simulink library "csc_ppc_phase_plane_ctrl_mtv_lib"  (R2014b)
settings: Solver=ode45  StartTime=0.0  StopTime=10.0  RelTol=1e-3
libraries: util_common_lib x2, util_quat_lib x2, util_info_lib x1, csc_cac_coarse_acs_cntrl_mtv_lib x1, csc_vac_vernier_acs_ctrl_lib x1
settings Model: Creator=tgorton  LastModifiedBy=tgorton

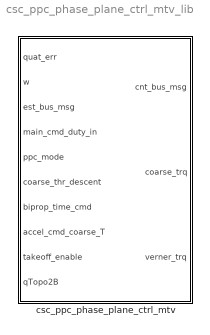
== system csc_ppc_phase_plane_ctrl_mtv_lib ==
  csc_ppc_phase_plane_ctrl_mtv : Subsystem

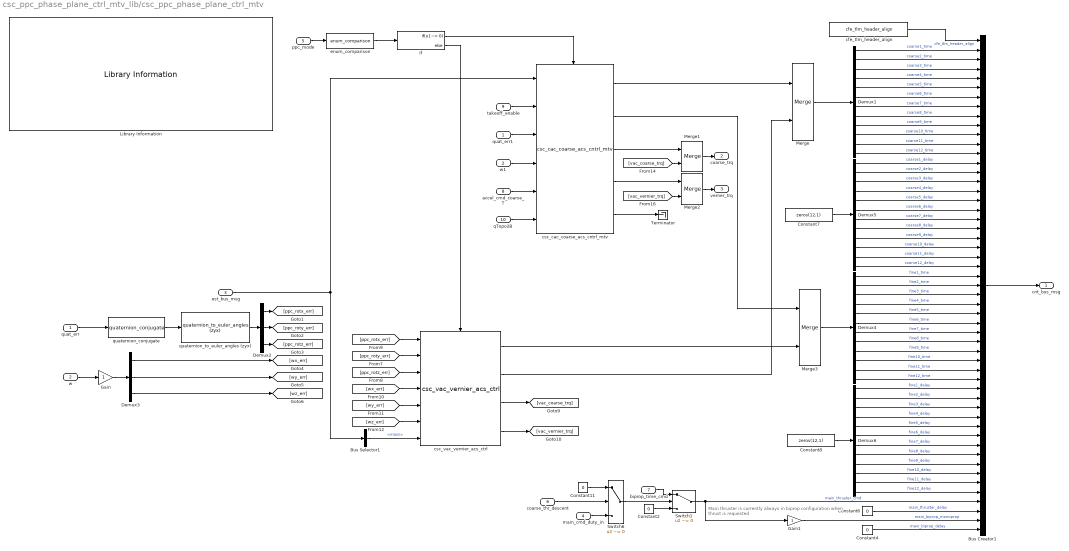
== system csc_ppc_phase_plane_ctrl_mtv_lib/csc_ppc_phase_plane_ctrl_mtv ==
  note: Main thruster is currently always in biprop configuration
      | when thrust is requested
  quat_err : Inport
  w : Inport  Port=2
  est_bus_msg : Inport  Port=3
  main_cmd_duty_in : Inport  Port=4
  ppc_mode : Inport  Port=5
  coarse_thr_descent : Inport  Port=6
  biprop_time_cmd : Inport  Port=7
  accel_cmd_coarse_T : Inport  Port=8
  takeoff_enable : Inport  Port=9
  qTopo2B : Inport  Port=10
  Bus Creator1 : BusCreator  Inputs=53  OutDataTypeStr=Bus: cnt_bus_msg  NonVirtualBus=on
  Bus Selector1 : BusSelector  OutputSignals=mass
  Constant11 : Constant  Value=0  OutDataTypeStr=boolean
  Constant2 : Constant  Value=0  OutDataTypeStr=uint8
  Constant4 : Constant  Value=0  OutDataTypeStr=uint8
  Constant6 : Constant  Value=0  OutDataTypeStr=uint8
  Constant7 : Constant  Value=zeros(12,1)  OutDataTypeStr=uint8
  Constant8 : Constant  Value=zeros(12,1)  OutDataTypeStr=uint8
  Demux{1,4..6} (4 alike) : Demux  Outputs=12
  Demux2 : Demux  Outputs=3
  Demux3 : Demux  Outputs=3
  Gain : Gain
  Gain1 : Gain  OutDataTypeStr=uint8
  If : If  IfExpression=u1~= 0
  Library Information : util_info_lib/Library Information  owner='jkaidy'
  Merge{,1..3} (4 alike) : Merge
  Switch1 : Switch  Criteria=u2 ~= 0
  Switch6 : Switch  Criteria=u2 ~= 0
  Terminator : Terminator
  cfe_tlm_header_align : util_common_lib/cfe_tlm_header_align
  csc_cac_coarse_acs_cntrl_mtv : csc_cac_coarse_acs_cntrl_mtv_lib/csc_cac_coarse_acs_cntrl_mtv
  csc_vac_vernier_acs_ctrl : csc_vac_vernier_acs_ctrl_lib/csc_vac_vernier_acs_ctrl
  enum_comparison : util_common_lib/enum_comparison  comparison_type===
  quat_err1 : InportShadow
  quaternion_conjugate : util_quat_lib/quaternion_conjugate  SystemSampleTime=-1
  quaternion_to_euler_angles (zyx) : util_quat_lib/quaternion_to_euler_angles (zyx)  SystemSampleTime=-1
  w1 : InportShadow  Port=2
  cnt_bus_msg : Outport
  coarse_trq : Outport  Port=2
  verner_trq : Outport  Port=3
  wires:
  quat_err1/1 -> csc_cac_coarse_acs_cntrl_mtv/3
  qTopo2B/1 -> csc_cac_coarse_acs_cntrl_mtv/6
  accel_cmd_coarse_T/1 -> csc_cac_coarse_acs_cntrl_mtv/5
  w1/1 -> csc_cac_coarse_acs_cntrl_mtv/4
  Bus Selector1/1 -> csc_vac_vernier_acs_ctrl/7  "<mass>"
  csc_cac_coarse_acs_cntrl_mtv/1 -> Merge/1
  Demux3/3 -> [wz_err]
  Demux3/2 -> [wy_err]
  Demux3/1 -> [wx_err]
  Gain/1 -> Demux3/1
  est_bus_msg/1 -> Bus Selector1/1, csc_cac_coarse_acs_cntrl_mtv/1
  ppc_mode/1 -> enum_comparison/1
  [ppc_rotx_err] -> csc_vac_vernier_acs_ctrl/1
  [ppc_roty_err] -> csc_vac_vernier_acs_ctrl/2
  [ppc_rotz_err] -> csc_vac_vernier_acs_ctrl/3
  [wz_err] -> csc_vac_vernier_acs_ctrl/6
  [wx_err] -> csc_vac_vernier_acs_ctrl/4
  [wy_err] -> csc_vac_vernier_acs_ctrl/5
  w/1 -> Gain/1
  quat_err/1 -> quaternion_conjugate/1
  biprop_time_cmd/1 -> Switch1/1
  Constant2/1 -> Switch1/3
  coarse_thr_descent/1 -> Switch6/2
  main_cmd_duty_in/1 -> Switch6/3
  Constant11/1 -> Switch6/1
  Switch6/1 -> Switch1/2
  Switch1/1 -> Bus Creator1/50, Gain1/1  "main_thruster_cmd"
  Bus Creator1/1 -> cnt_bus_msg/1
  quaternion_to_euler_angles (zyx)/1 -> Demux2/1
  quaternion_conjugate/1 -> quaternion_to_euler_angles (zyx)/1
  Demux2/1 -> [ppc_rotx_err]
  Demux2/3 -> [ppc_rotz_err]
  Demux2/2 -> [ppc_roty_err]
  enum_comparison/1 -> If/1
  If/1 -> csc_cac_coarse_acs_cntrl_mtv/Action
  If/2 -> csc_vac_vernier_acs_ctrl/Action
  Merge1/1 -> coarse_trq/1
  csc_cac_coarse_acs_cntrl_mtv/3 -> Merge1/1
  Merge2/1 -> verner_trq/1
  csc_cac_coarse_acs_cntrl_mtv/4 -> Merge2/1
  csc_vac_vernier_acs_ctrl/3 -> [vac_coarse_trq]
  [vac_coarse_trq] -> Merge1/2
  [vac_vernier_trq] -> Merge2/2
  cfe_tlm_header_align/1 -> Bus Creator1/1  "cfe_tlm_header_align"
  csc_vac_vernier_acs_ctrl/4 -> [vac_vernier_trq]
  csc_cac_coarse_acs_cntrl_mtv/2 -> Merge3/1
  Merge/1 -> Demux1/1
  Demux1/1 -> Bus Creator1/2  "coarse1_time"
  Demux1/8 -> Bus Creator1/9  "coarse8_time"
  Demux1/9 -> Bus Creator1/10  "coarse9_time"
  Demux1/12 -> Bus Creator1/13  "coarse12_time"
  Demux1/7 -> Bus Creator1/8  "coarse7_time"
  Demux1/4 -> Bus Creator1/5  "coarse4_time"
  Demux1/6 -> Bus Creator1/7  "coarse6_time"
  Demux1/3 -> Bus Creator1/4  "coarse3_time"
  Demux1/5 -> Bus Creator1/6  "coarse5_time"
  Demux1/10 -> Bus Creator1/11  "coarse10_time"
  Demux1/2 -> Bus Creator1/3  "coarse2_time"
  Demux1/11 -> Bus Creator1/12  "coarse11_time"
  Merge3/1 -> Demux4/1
  Demux5/3 -> Bus Creator1/16  "coarse3_delay"
  Demux5/4 -> Bus Creator1/17  "coarse4_delay"
  Demux5/6 -> Bus Creator1/19  "coarse6_delay"
  Demux5/8 -> Bus Creator1/21  "coarse8_delay"
  Demux5/2 -> Bus Creator1/15  "coarse2_delay"
  Demux5/12 -> Bus Creator1/25  "coarse12_delay"
  Demux5/9 -> Bus Creator1/22  "coarse9_delay"
  Demux5/5 -> Bus Creator1/18  "coarse5_delay"
  Demux5/1 -> Bus Creator1/14  "coarse1_delay"
  Demux5/11 -> Bus Creator1/24  "coarse11_delay"
  Demux5/7 -> Bus Creator1/20  "coarse7_delay"
  Demux5/10 -> Bus Creator1/23  "coarse10_delay"
  Demux4/4 -> Bus Creator1/29  "fine4_time"
  Demux4/9 -> Bus Creator1/34  "fine9_time"
  Demux4/10 -> Bus Creator1/35  "fine10_time"
  Demux4/8 -> Bus Creator1/33  "fine8_time"
  Demux4/7 -> Bus Creator1/32  "fine7_time"
  Demux4/2 -> Bus Creator1/27  "fine2_time"
  Demux4/1 -> Bus Creator1/26  "fine1_time"
  Demux4/5 -> Bus Creator1/30  "fine5_time"
  Demux4/12 -> Bus Creator1/37  "fine12_time"
  Demux4/3 -> Bus Creator1/28  "fine3_time"
  Demux4/6 -> Bus Creator1/31  "fine6_time"
  Demux4/11 -> Bus Creator1/36  "fine11_time"
  Constant4/1 -> Bus Creator1/53  "main_biprop_delay"
  Constant6/1 -> Bus Creator1/51  "main_thruster_delay"
  Demux6/1 -> Bus Creator1/38  "fine1_delay"
  Demux6/10 -> Bus Creator1/47  "fine10_delay"
  Demux6/4 -> Bus Creator1/41  "fine4_delay"
  Demux6/9 -> Bus Creator1/46  "fine9_delay"
  Demux6/6 -> Bus Creator1/43  "fine6_delay"
  Demux6/3 -> Bus Creator1/40  "fine3_delay"
  Demux6/8 -> Bus Creator1/45  "fine8_delay"
  Demux6/5 -> Bus Creator1/42  "fine5_delay"
  Demux6/2 -> Bus Creator1/39  "fine2_delay"
  Demux6/12 -> Bus Creator1/49  "fine12_delay"
  Demux6/7 -> Bus Creator1/44  "fine7_delay"
  Demux6/11 -> Bus Creator1/48  "fine11_delay"
  Constant7/1 -> Demux5/1
  Constant8/1 -> Demux6/1
  csc_vac_vernier_acs_ctrl/1 -> Merge3/2
  csc_vac_vernier_acs_ctrl/2 -> Merge/2
  Gain1/1 -> Bus Creator1/52  "main_biprop_monoprop"
  csc_cac_coarse_acs_cntrl_mtv/5 -> Terminator/1
  takeoff_enable/1 -> csc_cac_coarse_acs_cntrl_mtv/2
